simulink model "ADRC_P3DX_WAOA"  (R2024b)
settings: Solver=FixedStepAuto  StartTime=0.0  StopTime=30  FixedStep=0.01  RelTol=1e-2
settings Model: Creator=Dell  LastModifiedBy=MMadi
settings DebuggingCC: AlgebraicLoopMsg=none  SigSpecEnsureSampleTimeMsg=none
settings RTWCC: GPUComputeCapability=3.5

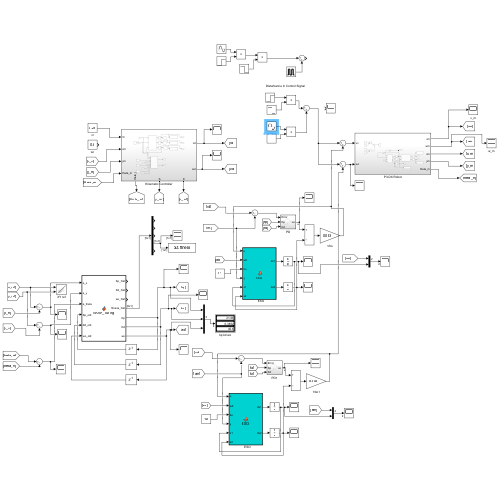
[thumbnail: Simulink's stored preview of the top-level diagram]
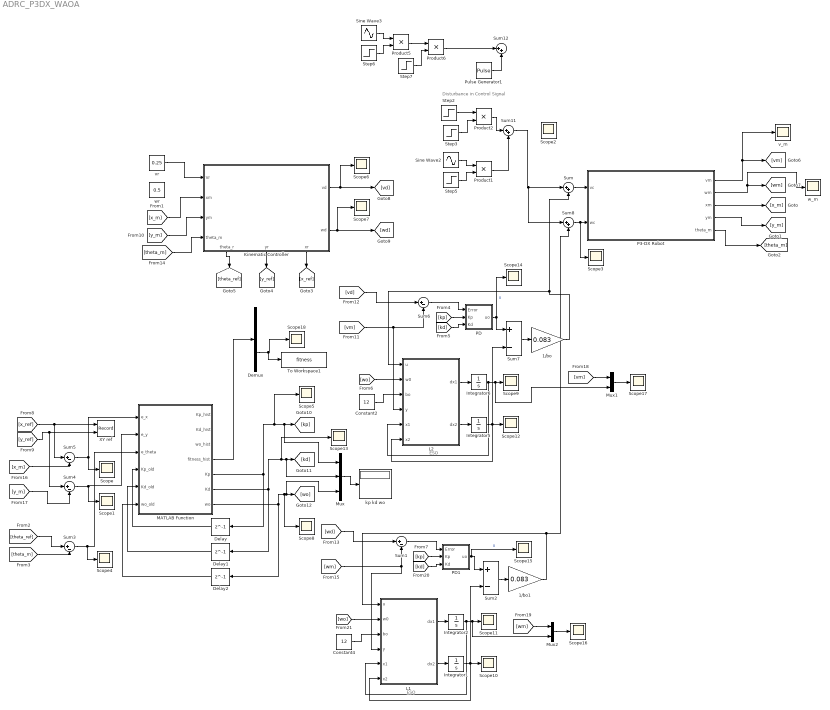
== system ADRC_P3DX_WAOA ==
  note: Disturbance in Control Signal
  note: ESO
  note: ESO
  1/bo : Gain  Gain=0.083
  1/bo1 : Gain  Gain=0.083
  Constant2 : Constant  Value=12
  Constant4 : Constant  Value=12
  Delay : Delay  DelayLength=1  InitialCondition=0
  Delay1 : Delay  DelayLength=1  InitialCondition=0
  Delay2 : Delay  DelayLength=1  InitialCondition=0
  Demux : Demux  Outputs=5
  Integrator{1..2,5..6} (4 alike) : Integrator
  Kinematic Controller : Subsystem
      settings: PortSchema="{\"entries\":[{\"content\":{\"sides\":[{\"content\":{\"connectorIds\":[\"In1\",\"In2\",\"In3\",\"In4\"]},\"type\":\"ConnectorPlacement.EquallySpacedRectSide\",\"uuid\":\"1dde3c4d-b362-4c98-bff5-173134d67a18\"},{\"content\":{\"connectorIds\":[\"Out1\",\"Out2\"],\"side\":\"RIGHT\"},\"type\":\"ConnectorPlacement.EquallySpacedRectSide\",\"uuid\":\"28a7b07a-1542-4ec6-930a-70e18e33702f\"},{\"content\":{\"side\":\"TOP\"},\"type\":\"ConnectorPlacement.EquallySpacedRectSide\",\"uuid\":\"fddfb50e-6b1f-4e7e-bd72-f809cd3d8285\"},{\"content\":{\"connectorIds\":[\"Out3\",\"Out4\",\"Out5\"],\"side\":\"BOTTOM\"},\"type\":\"ConnectorPlacement.EquallySpacedRectSide\",\"uuid\":\"0cbc9f95-9386-4a92-999a-6cc6855b0431\"}]},\"type\":\"ConnectorPlacement.EquallySpacedConnector\",\"uuid\":\"21383b85-61ab-4832-be46-2fedf08e757e\"}],\"packageUris\":[\"http://schema.mathworks.com/mf0/Connector/R2020b\"],\"version\":\"1.0\"}"
  L1 : MATLAB Function  TreatAsAtomicUnit=on
  L2 : MATLAB Function  TreatAsAtomicUnit=on
  MATLAB Function : MATLAB Function  TreatAsAtomicUnit=on
  Mux : Mux  Inputs=3
  Mux1 : Mux  Inputs=2
  Mux2 : Mux  Inputs=2
  P3-DX Robot : Subsystem
  PD : Subsystem
  PD1 : Subsystem
  Product{1..2,5..6} (4 alike) : Product
  Pulse Generator1 : DiscretePulseGenerator  PulseType=Time based  Amplitude=5  Period=1  PulseWidth=35  PhaseDelay=15
  Scope{,1..18} (19 alike) : Scope
  Sine Wave2 : Sin  Amplitude=4.2  Frequency=2  SampleTime=0
  Sine Wave3 : Sin  Amplitude=3.5  Frequency=2  SampleTime=0
  Step2 : Step  Time=8  After=2.1  SampleTime=0
  Step3 : Step  Time=10  Before=2.1  After=0  SampleTime=0
  Step5 : Step  Time=20  SampleTime=0
  Step6 : Step  Time=3.2  SampleTime=0
  Step7 : Step  Time=15  Before=1  After=0  SampleTime=0
  Sum{,8,11..12} (4 alike) : Sum  Inputs=|++
  Sum{1,3..6} (5 alike) : Sum  Inputs=|+-
  Sum2 : Sum  Inputs=+-
  Sum7 : Sum  Inputs=+-
  To Workspace1 : ToWorkspace  VariableName=fitness  SaveFormat=Timeseries  SampleTime=-1
  XY ref : Record  FileSettingsInternal="{\"entries\":[{\"content\":{\"excelSettings\":{\"content\":{},\"type\":\"Streamout.ExcelSettings\"}},\"type\":\"Streamout.FileSettingStorage\",\"uuid\":\"\"}],\"packageUris\":[\"http:\\/\\/schema.mathworks.com\\/mf0\\/streamout_blocks\\/R2020a\"],\"version\":\"1.0\"}"  Layout=[1 1]  SignalsInternal="{\"entries\":[{\"content\":{\"signals\":[{\"content\":{\"blockPath\":[],\"dimensions\":[1],\"domain\":\"\",\"lineColor\":\"#4dbeee\",\"lineWidth\":2,\"port\":1,\"signalID\":1,\"signalName\":\"From8\"},\"type\":\"RecordBlkView.Signal\",\"uuid\":\"\"},{\"content\":{\"blockPath\":[],\"dimensions\":[1],\"domain\":\"\",\"lineColor\":\"#a2142f\",\"lineWidth\":2,\"port\":2,\"signalID\":2,\"signalName\":\"From9\"},\"type\":\"RecordBlkView.Signal\",\"uuid\":\"\"}]},\"type\":\"RecordBlkView.InputSignals\",\"uuid\":\"\"}],\"packageUris\":[\"http:\\/\\/schema.mathworks.com\\/mf0\\/streamout_blocks\\/R2020a\"],\"version\":\"1.0\"}"  VisualizationBindings="{\"xyplotplugin\":{\"info\":[{\"series\":[],\"subplotID\":1}]}}"  CompatibilityTag=XY
  kp kd wo : Display
  v_m : Scope
  vr : Constant  Value=0.25
  w_m : Scope
  wr : Constant  Value=0.5
  wires:
  [y_ref] -> Sum4/1, XY ref/2
  [x_ref] -> Sum5/1, XY ref/1
  [y_m] -> Kinematic Controller/3(ym)
  vr/1 -> Kinematic Controller/1(Vr)
  [x_m] -> Kinematic Controller/2(xm)
  [theta_m] -> Kinematic Controller/4(theta_m)
  P3-DX Robot/3(xm) -> [x_m]
  P3-DX Robot/4(ym) -> [y_m]
  P3-DX Robot/5(theta_m) -> [theta_m]
  Kinematic Controller/5(xr) -> [x_ref]
  Kinematic Controller/4(yr) -> [y_ref]
  Kinematic Controller/3(theta_r) -> [theta_ref]
  Kinematic Controller/2(wd) -> [wd], Scope7/1
  Kinematic Controller/1(vd) -> [vd], Scope6/1
  1/bo/1 -> Sum/2, L2/1(u)
  [vd] -> Sum6/1
  Integrator6/1 -> L2/5(x1), Mux1/2, Scope9/1
  Sum7/1 -> 1/bo/1
  PD/1(uo) -> Sum7/1, Scope14/1  "u"
  [vm] -> Sum6/2, L2/4(y)
  Sum6/1 -> PD/1(Error)
  Integrator5/1 -> Sum7/2, Scope12/1, L2/6(x2)
  L2/2(dx2) -> Integrator5/1
  L2/1(dx1) -> Integrator6/1
  L1/2(dx2) -> Integrator1/1
  Integrator1/1 -> Sum2/2, Scope10/1, L1/6(x2)
  [wm] -> L1/4(y), Sum1/2
  Sum1/1 -> PD1/1(Error)
  Sum2/1 -> 1/bo1/1
  Integrator2/1 -> L1/5(x1), Mux2/2, Scope11/1
  L1/1(dx1) -> Integrator2/1
  [wd] -> Sum1/1
  Constant4/1 -> L1/3(bo)
  PD1/1(uo) -> Scope15/1, Sum2/1  "u"
  1/bo1/1 -> Sum8/2, L1/1(u)
  Sum/1 -> P3-DX Robot/1(vc)
  Sum8/1 -> Scope3/1, P3-DX Robot/2(wc)
  [vm] -> Mux1/1
  Mux1/1 -> Scope17/1
  [wm] -> Mux2/1
  Mux2/1 -> Scope16/1
  Constant2/1 -> L2/3(bo)
  Sine Wave2/1 -> Product1/1
  Step5/1 -> Product1/2
  Step3/1 -> Product2/2
  Step2/1 -> Product2/1
  P3-DX Robot/1(vm) -> v_m/1, [vm]
  P3-DX Robot/2(wm) -> w_m/1, [wm]
  MATLAB Function/6(Kd) -> Scope13/1, Mux/2, [kd], Delay1/1
  MATLAB Function/7(wo) -> Scope8/1, Mux/3, [wo], Delay2/1
  MATLAB Function/5(Kp) -> Scope5/1, Mux/1, [kp], Delay/1
  [theta_ref] -> Sum3/1
  [theta_m] -> Sum3/2
  [y_m] -> Sum4/2
  [x_m] -> Sum5/2
  Sum5/1 -> Scope/1, MATLAB Function/1(e_x)
  Sum4/1 -> Scope1/1, MATLAB Function/2(e_y)
  Sum3/1 -> Scope4/1, MATLAB Function/3(e_theta)
  [kp] -> PD/2(Kp)
  [kd] -> PD/3(Kd)
  [wo] -> L2/2(w0)
  Delay/1 -> MATLAB Function/4(Kp_old)
  Delay1/1 -> MATLAB Function/5(Kd_old)
  Delay2/1 -> MATLAB Function/6(wo_old)
  Mux/1 -> kp kd wo/1
  [kp] -> PD1/2(Kp)
  [kd] -> PD1/3(Kd)
  [wo] -> L1/2(w0)
  Product1/1 -> Sum11/2
  Product2/1 -> Sum11/1
  Product5/1 -> Product6/1
  Step7/1 -> Product6/2
  Sine Wave3/1 -> Product5/1
  Product6/1 -> Sum12/1
  Pulse Generator1/1 -> Sum12/2
  Step6/1 -> Product5/2
  Demux/4 -> To Workspace1/1, Scope18/1
  MATLAB Function/4(fitness_hist) -> Demux/1
  Sum11/1 -> Sum8/1, Sum/1

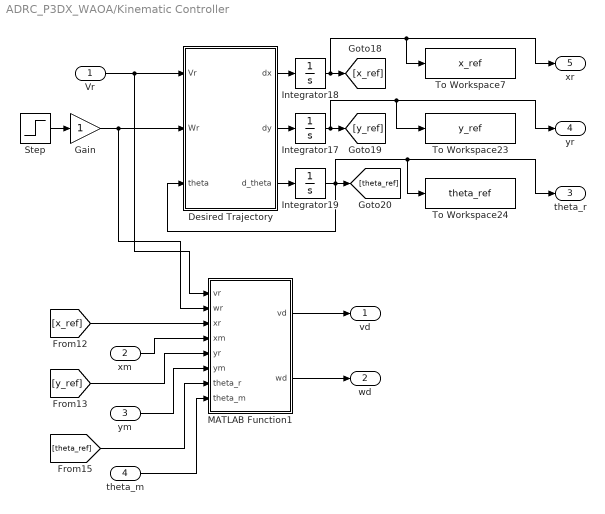
== system ADRC_P3DX_WAOA/Kinematic Controller ==
  Vr : Inport
  xm : Inport  Port=2
  ym : Inport  Port=3
  theta_m : Inport  Port=4
  " Desired Trajectory" : MATLAB Function  TreatAsAtomicUnit=on
  Gain : Gain
  Integrator17 : Integrator  InitialCondition=-0.5
  Integrator18 : Integrator
  Integrator19 : Integrator
  MATLAB Function1 : MATLAB Function  TreatAsAtomicUnit=on
  Step : Step  Time=16  Before=0.5  After=0.4  SampleTime=0
  To Workspace23 : ToWorkspace  VariableName=y_ref  SaveFormat=Timeseries  SampleTime=-1
  To Workspace24 : ToWorkspace  VariableName=theta_ref  SaveFormat=Timeseries  SampleTime=-1
  To Workspace7 : ToWorkspace  VariableName=x_ref  SaveFormat=Timeseries  SampleTime=-1
  vd : Outport
  wd : Outport  Port=2
  theta_r : Outport  Port=3
  yr : Outport  Port=4
  xr : Outport  Port=5
  wires:
  " Desired Trajectory"/3(d_theta) -> Integrator19/1
  Integrator19/1 -> theta_r/1, To Workspace24/1, " Desired Trajectory"/3(theta), [theta_ref]
  Integrator18/1 -> xr/1, To Workspace7/1, [x_ref]
  Vr/1 -> MATLAB Function1/1(vr), " Desired Trajectory"/1(Vr)
  " Desired Trajectory"/1(dx) -> Integrator18/1
  Gain/1 -> MATLAB Function1/2(wr), " Desired Trajectory"/2(Wr)
  MATLAB Function1/1(vd) -> vd/1
  MATLAB Function1/2(wd) -> wd/1
  " Desired Trajectory"/2(dy) -> Integrator17/1
  Integrator17/1 -> yr/1, To Workspace23/1, [y_ref]
  [x_ref] -> MATLAB Function1/3(xr)
  xm/1 -> MATLAB Function1/4(xm)
  [y_ref] -> MATLAB Function1/5(yr)
  ym/1 -> MATLAB Function1/6(ym)
  [theta_ref] -> MATLAB Function1/7(theta_r)
  theta_m/1 -> MATLAB Function1/8(theta_m)
  Step/1 -> Gain/1

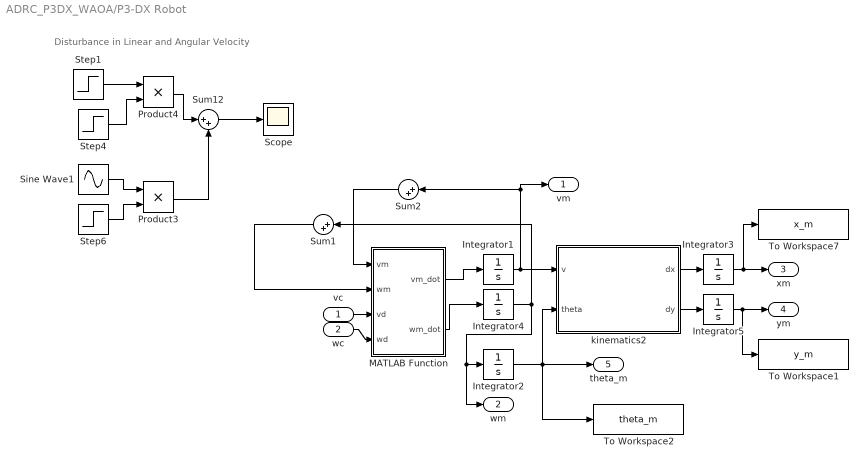
== system ADRC_P3DX_WAOA/P3-DX Robot ==
  note: Disturbance in Linear and Angular Velocity
  vc : Inport
  wc : Inport  Port=2
  Integrator{1..5} (5 alike) : Integrator
  MATLAB Function : MATLAB Function  TreatAsAtomicUnit=on
  Product3 : Product
  Product4 : Product
  Scope : Scope
  Sine Wave1 : Sin  Amplitude=4  Frequency=2  SampleTime=0
  Step1 : Step  Time=8  After=2.2  SampleTime=0
  Step4 : Step  Time=10  Before=2.2  After=0  SampleTime=0
  Step6 : Step  Time=20  SampleTime=0
  Sum1 : Sum  Inputs=|++
  Sum12 : Sum  Inputs=|++
  Sum2 : Sum  Inputs=|++
  To Workspace1 : ToWorkspace  VariableName=y_m  SaveFormat=Timeseries  SampleTime=-1
  To Workspace2 : ToWorkspace  VariableName=theta_m  SaveFormat=Timeseries  SampleTime=-1
  To Workspace7 : ToWorkspace  VariableName=x_m  SaveFormat=Timeseries  SampleTime=-1
  kinematics2 : MATLAB Function  TreatAsAtomicUnit=on
  vm : Outport
  wm : Outport  Port=2
  xm : Outport  Port=3
  ym : Outport  Port=4
  theta_m : Outport  Port=5
  wires:
  Integrator2/1 -> To Workspace2/1, theta_m/1, kinematics2/2(theta)
  MATLAB Function/1(vm_dot) -> Integrator1/1
  MATLAB Function/2(wm_dot) -> Integrator4/1
  Integrator1/1 -> kinematics2/1(v), Sum2/1, vm/1
  Integrator3/1 -> To Workspace7/1, xm/1
  Integrator4/1 -> Integrator2/1, wm/1, Sum1/1
  kinematics2/2(dy) -> Integrator5/1
  vc/1 -> MATLAB Function/3(vd)
  kinematics2/1(dx) -> Integrator3/1
  wc/1 -> MATLAB Function/4(wd)
  Integrator5/1 -> To Workspace1/1, ym/1
  Product4/1 -> Sum12/1
  Step4/1 -> Product4/2
  Step1/1 -> Product4/1
  Product3/1 -> Sum12/2
  Sine Wave1/1 -> Product3/1
  Step6/1 -> Product3/2
  Sum1/1 -> MATLAB Function/2(wm)
  Sum2/1 -> MATLAB Function/1(vm)
  Sum12/1 -> Scope/1

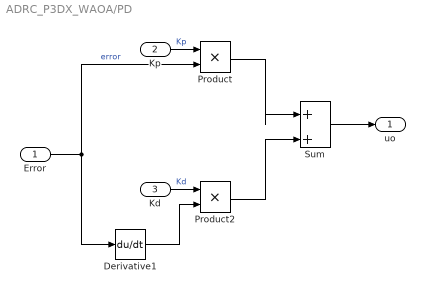
== system ADRC_P3DX_WAOA/PD ==
  Error : Inport
  Kp : Inport  Port=2
  Kd : Inport  Port=3
  Derivative1 : Derivative
  Product : Product
  Product2 : Product
  Sum : Sum  Inputs=|++
  uo : Outport
  wires:
  Derivative1/1 -> Product2/2
  Sum/1 -> uo/1
  Product/1 -> Sum/1
  Error/1 -> Derivative1/1, Product/2  "error"
  Kd/1 -> Product2/1  "Kd"
  Kp/1 -> Product/1  "Kp"
  Product2/1 -> Sum/2

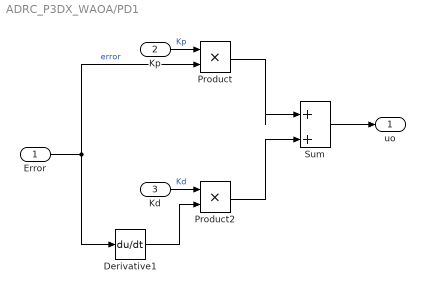
== system ADRC_P3DX_WAOA/PD1 ==
  Error : Inport
  Kp : Inport  Port=2
  Kd : Inport  Port=3
  Derivative1 : Derivative
  Product : Product
  Product2 : Product
  Sum : Sum  Inputs=|++
  uo : Outport
  wires:
  Derivative1/1 -> Product2/2
  Sum/1 -> uo/1
  Product/1 -> Sum/1
  Error/1 -> Derivative1/1, Product/2  "error"
  Kd/1 -> Product2/1  "Kd"
  Kp/1 -> Product/1  "Kp"
  Product2/1 -> Sum/2

== matlab function ADRC_P3DX_WAOA/L2 ==
  data: dx1 output; dx2 output; u input; w0 input; bo input; y input; x1 input; x2 input
function [dx1, dx2] = ESO(u, w0,bo, y, x1, x2)

%bo=[15.5311 -3.5587;
    %-3.5587 15.5311];
% l1, l2, l3 ARE THE OBSERVER GAINS IN ESO calcualated using w0
L1=2*w0;   
L2=w0^2;

e = x1-y;

dx1 = x2 + (bo * u) - (L1 * e);
dx2 = - (L2 * e);

== matlab function ADRC_P3DX_WAOA/Kinematic Controller/ Desired Trajectory ==
  data: Vr input; Wr input; theta input; dx output; dy output; d_theta output
function [dx, dy, d_theta] = desiredtraj(Vr, Wr, theta)
    dx = cos(theta) * Vr ;
    dy = sin(theta) * Vr ;
    d_theta = Wr;
    

end

== matlab function ADRC_P3DX_WAOA/Kinematic Controller/MATLAB Function1 ==
  data: vr input; wr input; xr input; vd output; xm input; yr input; ym input; theta_r input; theta_m input; wd output
function [vd, wd] = fcn(vr, wr, xr, xm, yr, ym, theta_r, theta_m)
ex = ((xr - xm) * cos(theta_m)) + ((yr - ym) * sin(theta_m));
ey = - ((xr - xm) * sin(theta_m)) + ((yr - ym) * cos(theta_m));

etheta = theta_r - theta_m;

kx = 0.8;
ky = 0.8;
kth = 0.8;

vd = (kx * ex) + (vr * cos(etheta));
wd = (ky * vr * ey ) + wr + (kth * sin(etheta));

== matlab function ADRC_P3DX_WAOA/P3-DX Robot/MATLAB Function ==
  data: vm input; vm_dot output; wm input; wm_dot output; vd input; wd input
function[vm_dot, wm_dot] = fcn(vm,wm,vd,wd)
k1 = 0.24089;
k2 = 0.2424;
k3 = -0.00093603;
k4 = 0.99629;
k5 = -0.0057256;
k6 = 1;


vm_dot = ((k3/k1) * (wm*wm)) - ((k4/k1) * vm) + (vd/k1);
wm_dot = - ((k5/k2) * (vm*wm)) - ((k6/k2) * wm) + (wd/k2);

== matlab function ADRC_P3DX_WAOA/P3-DX Robot/kinematics2 ==
  data: v input; dx output; dy output; theta input
function [dx, dy] = kinematics(v, theta)


dx =  v .* cos(theta);
dy =  v .* sin(theta);

== matlab function ADRC_P3DX_WAOA/L1 ==
  data: dx1 output; dx2 output; u input; w0 input; bo input; y input; x1 input; x2 input
function [dx1,dx2] =ESO(u,w0,bo, y, x1,x2)
%bo=[15.5311 -3.5587;
    %-3.5587 15.5311];
% l1, l2, l3 ARE THE OBSERVER GAINS IN ESO calcualated using w0
L1=2*w0;   
L2=w0^2;

e = x1-y;

dx1 = x2 + (bo * u) - (L1 * e);
dx2 = - (L2 * e);

== matlab function ADRC_P3DX_WAOA/MATLAB Function ==
  settings: updateMethod=DISCRETE
  data: Kp_hist output; Kd_hist output; wo_hist output; fitness_hist output; e_x input; Kp output; e_y input; e_theta input; Kp_old input; Kd_old input; wo_old input; Kd output; wo output

function [Kp_hist, Kd_hist, wo_hist, fitness_hist, Kp, Kd, wo] = WAOA_Tuning(e_x, e_y, e_theta, Kp_old, Kd_old, wo_old)

    % Parameters
    num_generations = 10;
    pop_size = 10;
    dim = 3; % [Kp, Kd, wo]
    lb = [0, 0, 0];
    ub = [100, 1, 50];

    % Fitness function (currently independent of Kp/Kd/wo - placeholder)
    fitness = @(params) sum(e_x.^2 + e_y.^2 + e_theta.^2);

    % Initialize population matrix
    X = zeros(pop_size, dim);
    for i = 1:dim
        X(:,i) = lb(i) + rand(pop_size,1).*(ub(i)-lb(i));
    end

    % Initialize fitness values
    fit = zeros(pop_size, 1);
    for i = 1:pop_size
        L = X(i,:);
        fit(i) = fitness(L);
    end

    % Initialize best fitness and solution
    [fbest, bestIdx] = min(fit);
    Xbest = X(bestIdx, :);

    % Initialize logs
    Kp_hist = zeros(num_generations, 1);
    Kd_hist = zeros(num_generations, 1);
    wo_hist = zeros(num_generations, 1);
    fitness_hist = zeros(num_generations, 1);

    % Main loop
    for t = 1:num_generations
        SW = Xbest;  % strongest walrus (best known solution)

        for i = 1:pop_size
            %% Phase 1: Feeding Strategy (Exploration)
            I = round(1 + rand());
            X_P1 = X(i,:) + rand(1,dim) .* (SW - I * X(i,:));
            X_P1 = max(min(X_P1, ub), lb);

            F_P1 = fitness(X_P1);
            if F_P1 < fit(i)
                X(i,:) = X_P1;
                fit(i) = F_P1;
            end

            %% Phase 2: Migration
            I = round(1 + rand());
            K = randperm(pop_size);
            K(K == i) = [];
            X_K = X(K(1),:);
            F_RAND = fit(K(1));

            if fit(i) > F_RAND
                X_P2 = X(i,:) + rand() * (X_K - I * X(i,:));
            else
                X_P2 = X(i,:) + rand() * (X(i,:) - X_K);
            end

            X_P2 = max(min(X_P2, ub), lb);
            F_P2 = fitness(X_P2);
            if F_P2 < fit(i)
                X(i,:) = X_P2;
                fit(i) = F_P2;
            end

            %% Phase 3: Escaping & Fighting Against Predators (Exploitation)
            LO_LOCAL = lb ./ t;
            HI_LOCAL = ub ./ t;
            X_P3 = X(i,:) + LO_LOCAL + rand() * (HI_LOCAL - LO_LOCAL);
            X_P3 = max(min(X_P3, ub), lb);

            F_P3 = fitness(X_P3);
            if F_P3 < fit(i)
                X(i,:) = X_P3;
                fit(i) = F_P3;
            end
        end

        % Update best solution of the current generation
        [curr_best, curr_bestIdx] = min(fit);
        if curr_best < fbest
            fbest = curr_best;
            Xbest = X(curr_bestIdx, :);
        end

        % Record history
        Kp_hist(t) = Xbest(1);
        Kd_hist(t) = Xbest(2);
        wo_hist(t) = Xbest(3);
        fitness_hist(t) = fbest;
    end

    % Final best parameters
    Kp = Xbest(1);
    Kd = Xbest(2);
    wo = Xbest(3);
end
